simulink model "MDSC_PLL"  (R2018b)
settings: Solver=VariableStepAuto  StartTime=0.0  StopTime=10.0  RelTol=1e-3
libraries: simulink x1, powerlib_meascontrol x1, powerlib x1
(part 1 of 2)
settings Model: Creator=lokes  LastModifiedBy=lokes

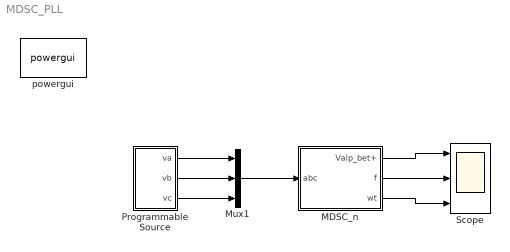
== system MDSC_PLL ==
  MDSC_n : Subsystem  mask{n=15, s=4, hr=1}
      mask prompts: n "MDSC Number (n)"; s "Selector (s): 1 for n= 6, 2 for n=9, 3 for n=12 and 4 for n=15"; hr "Required Component Extraction (hr)"
  Mux1 : Mux  Inputs=3
  Programmable Source : Subsystem  mask(CDSC - PLL){f=50, V=230}
      mask prompts: f "Fundamental grid frequency (f) in Hz"; V "Fundamental grid voltage (V) in RMS volts"
      mask help: Programmable source generates a signal with fundamental and odd harmonic signals upto 13th frequency component.
  Scope : Scope  NumInputPorts=3
  powergui : powerlib/powergui  Priority=1  SimulationMode=Discrete  SampleTime=10e-6  frequency=60  Iterations=50  frequencyindice=60  Pbase=100e6  ErrMax=1e-4  UnitsV=kV  UnitsW=MW  buscounter=0  FunctionMessages=off  echomessages=off  EnableUseOfTLC=off  CurrentSourceSwitches=off  DisableSnubberDevices=off  DisableRonSwitches=off  DisableVfSwitches=off  DisplayEquations=off  SolverType=Tustin  Interpol=off  ExternalGateDelay=off  methode=off  Ts=0  x0status=blocks  SPID=off  SwTol=0  HookPort=off  RestoreLinks=warning  ResistiveCurrentMeasurement=off  Frange=[0:2:500]  Ylog=off  Xlog=on  ShowGrid=off  save=off  variable=ZData  structure=0  ZoomFFT=off  StartTime=0.0  cycles=1  DisplayStyle=1  fundamental=60  FreqAxis=off  MaxFrequency=1000  frequencyindicesteady=1  RmsSteady=1  display=off
      settings: SourceProductName=Simscape Electrical
  wires:
  Programmable Source/1(va) -> Mux1/1
  Programmable Source/2(vb) -> Mux1/2
  Programmable Source/3(vc) -> Mux1/3
  Mux1/1 -> MDSC_n/1(abc)
  MDSC_n/1(Valp_bet+) -> Scope/1
  MDSC_n/2(f) -> Scope/2
  MDSC_n/3(wt) -> Scope/3

== system MDSC_PLL/MDSC_n ==
  abc : Inport
  3 : Constant  Value=0
  Demux : Demux  Outputs=3
  MDSC_n : Subsystem
  Mux6 : Mux  Inputs=2
  Mux7 : Mux  Inputs=2
  SRF-PLL1 : Subsystem
  abc to alpha-beta-Zero : Subsystem
      mask Display:
      | plot([0 1], [0,1])
      | text(0.15,0.7,'abc')
      | text(0.55, 0.3,'\alpha\beta0','texmode','on')
  Valp_bet+ : Outport
  f : Outport  Port=2
  wt : Outport  Port=3
  tag scope: f_pll_m3=global
  wires:
  abc/1 -> abc to alpha-beta-Zero/1(abc)
  abc to alpha-beta-Zero/1(al_be_0) -> Demux/1
  Demux/1 -> MDSC_n/1(Alpha)
  Demux/2 -> MDSC_n/2(Beta)
  MDSC_n/1(MDSC_n_alp) -> Mux6/1
  MDSC_n/2(MDSC_n_Bet) -> Mux6/2
  Mux6/1 -> Valp_bet+/1, Mux7/1
  3/1 -> Mux7/2
  Mux7/1 -> SRF-PLL1/1(al-be-0)
  SRF-PLL1/1(f) -> f/1, [f_pll_m3]
  SRF-PLL1/2(wt) -> wt/1

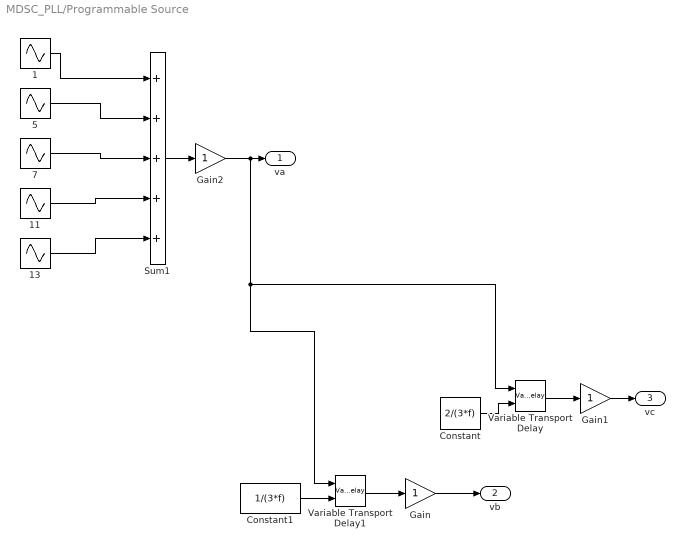
== system MDSC_PLL/Programmable Source ==
  1 : Sin  Amplitude=V*sqrt(2)  Frequency=2*pi*f  Phase=0*pi/2  SampleTime=0
  11 : Sin  Amplitude=V*sqrt(2)/11  Frequency=2*pi*11*f  Phase=0*pi/2  SampleTime=0
  13 : Sin  Amplitude=V*sqrt(2)/13  Frequency=2*pi*13*f  Phase=0*pi/2  SampleTime=0
  5 : Sin  Amplitude=V*sqrt(2)/5  Frequency=2*pi*5*f  Phase=0*pi/2  SampleTime=0
  7 : Sin  Amplitude=V*sqrt(2)/7  Frequency=2*pi*7*f  Phase=0*pi/2  SampleTime=0
  Constant : Constant  Value=2/(3*f)
  Constant1 : Constant  Value=1/(3*f)
  Gain : Gain
  Gain1 : Gain
  Gain2 : Gain
  Sum1 : Sum  Inputs=+++++
  Variable Transport Delay : VariableTransportDelay  VariableDelayType=Variable transport delay  MaximumDelay=10
  Variable Transport Delay1 : VariableTransportDelay  VariableDelayType=Variable transport delay  MaximumDelay=10
  va : Outport
  vb : Outport  Port=2
  vc : Outport  Port=3
  wires:
  Constant1/1 -> Variable Transport Delay1/2
  Constant/1 -> Variable Transport Delay/2
  Variable Transport Delay1/1 -> Gain/1
  Variable Transport Delay/1 -> Gain1/1
  Gain/1 -> vb/1
  Gain1/1 -> vc/1
  Sum1/1 -> Gain2/1
  Gain2/1 -> Variable Transport Delay1/1, Variable Transport Delay/1, va/1
  1/1 -> Sum1/1
  5/1 -> Sum1/2
  7/1 -> Sum1/3
  11/1 -> Sum1/4
  13/1 -> Sum1/5

== system MDSC_PLL/MDSC_n/MDSC_n ==
  Alpha : Inport
  Beta : Inport  Port=2
  DSC_Beta : Subsystem
  DSC_alpha : Subsystem
  MDSC_n_alp : Outport
  MDSC_n_Bet : Outport  Port=2
  wires:
  DSC_alpha/1(Out) -> MDSC_n_alp/1
  DSC_Beta/1(Out) -> MDSC_n_Bet/1
  Alpha/1 -> DSC_Beta/1(Alpha), DSC_alpha/1(Alpha)
  Beta/1 -> DSC_Beta/2(Beta), DSC_alpha/2(Beta)

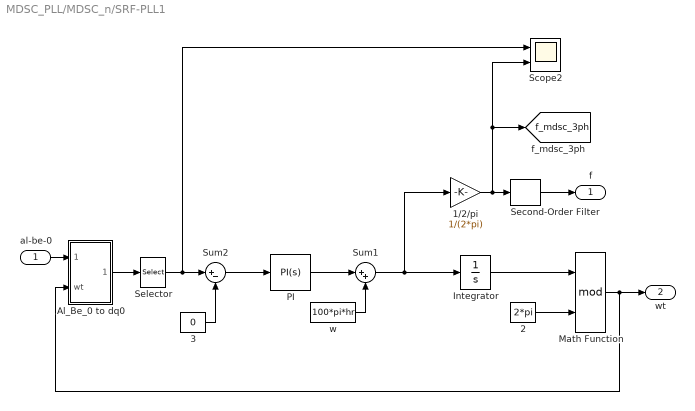
== system MDSC_PLL/MDSC_n/SRF-PLL1 ==
  al-be-0 : Inport
  1/2/pi : Gain  Gain=1/(2*pi)
  2 : Constant  Value=2*pi
  3 : Constant  Value=0
  Al_Be_0 to dq0 : Subsystem
      mask Display:
      | plot([0 1], [0,1])
      | port_label('input', 1, '\alpha\beta0','texmode','on')
      | port_label('input', 2, 'wt')
      | port_label('output', 1, 'dq0')
  Integrator : Integrator
  Math Function : Math  Operator=mod  SaturateOnIntegerOverflow=on
  "PI " : simulink/Continuous/PID Controller  Controller=PI  Form=Parallel  TimeDomain=Continuous-time  SampleTime=100e-6  IntegratorMethod=Forward Euler  FilterMethod=Forward Euler  ControllerParametersSource=internal  P=10  I=30  D=0  UseFilter=on  N=100  TunerSelectOption=Transfer Function Based (PID Tuner App)  InitialConditionSource=internal  InitialConditionForIntegrator=0  InitialConditionForFilter=0  DifferentiatorICPrevScaledInput=0  ExternalReset=none  TrackingMode=off  Kt=1  LimitOutput=off  UpperSaturationLimit=inf  LowerSaturationLimit=-inf  LinearizeAsGain=on  AntiWindupMode=none  Kb=1  POutMin=[]  POutMax=[]  IOutMin=[]  IOutMax=[]  DOutMin=[]  DOutMax=[]  NOutMin=[]  NOutMax=[]  SumOutMin=[]  SumOutMax=[]  SaturationOutMin=[]  SaturationOutMax=[]  PParamMin=[]  PParamMax=[]  IParamMin=[]  IParamMax=[]  DParamMin=[]  DParamMax=[]  NParamMin=[]  NParamMax=[]  KbParamMin=[]  KbParamMax=[]  KtParamMin=[]  KtParamMax=[]  KbOutMin=[]  KbOutMax=[]  KtOutMin=[]  KtOutMax=[]  IntegratorOutMin=[]  IntegratorOutMax=[]  FilterOutMin=[]  FilterOutMax=[]  SumI1OutMin=[]  SumI1OutMax=[]  SumI2OutMin=[]  SumI2OutMax=[]  SumI3OutMin=[]  SumI3OutMax=[]  SumI4OutMin=[]  SumI4OutMax=[]  SumDOutMin=[]  SumDOutMax=[]  DifferentiatorOutMin=[]  DifferentiatorOutMax=[]  FilterDiffOutCoefMin=[]  FilterDiffOutCoefMax=[]  ReciprocalOutMin=[]  ReciprocalOutMax=[]  SumDenOutMin=[]  SumDenOutMax=[]  SumNumOutMin=[]  SumNumOutMax=[]  DivideOutMin=[]  DivideOutMax=[]  IntegratorContinuousStateAttributes=''  IntegratorStateMustResolveToSignalObject=off  IntegratorRTWStateStorageClass=Auto  FilterContinuousStateAttributes=''  FilterStateMustResolveToSignalObject=off  FilterRTWStateStorageClass=Auto  ParallelPVariant=InternalParameters  IdealPVariant=Disabled  IVariant=InternalParameters  DVariant=Disabled  IntegratorVariant=Continuous  SatVariant=Disabled  AWVariant=Passthrough  PCopyVariant=Disabled  TRVariant=Disabled  FdbkBlocksVariant=Forward  IdealPFdbkVariant=Disabled  SatFdbkVariant=Disabled  DerivativeFilterVariant=Disabled  NVariant=Disabled  NCopyVariant=Disabled_SignalSpec  FilterICVariant=Disabled  IntegratorICVariant=InternalICs  ExternalResetVariant=Disabled  TRSumVariant=Passthrough  SumFdbkVariant=Disabled  SumVariant=Sum_PI
  Scope2 : Scope  NumInputPorts=2
  Second-Order Filter : powerlib_meascontrol/Filters/Second-Order Filter  FilterType=Lowpass  Fo=5  Zeta=0.707  Ts=0  Initialize=off  Vac_Init="[0,  0,  50]"  Vdc_Init=0  PlotResponse=off  FreqRange=[0, 500, 1]
      settings: SourceProductName=Simscape Electrical  SourceProductBaseCode=PS
  Selector : Selector  InputPortWidth=3  IndexOptions=Index vector (dialog)  Indices=1  OutputSizes=1
  Sum1 : Sum  Inputs=|++
  Sum2 : Sum  Inputs=|+-
  w : Constant  Value=100*pi*hr
  f : Outport
  wt : Outport  Port=2
  tag scope: f_mdsc_3ph=global
  wires:
  1/2/pi/1 -> Second-Order Filter/1, [f_mdsc_3ph], Scope2/2
  Math Function/1 -> Al_Be_0 to dq0/2(wt), wt/1
  Integrator/1 -> Math Function/1
  2/1 -> Math Function/2
  Sum1/1 -> Integrator/1, 1/2/pi/1
  w/1 -> Sum1/2
  "PI "/1 -> Sum1/1
  Sum2/1 -> "PI "/1
  al-be-0/1 -> Al_Be_0 to dq0/1(Al_Be_0)
  3/1 -> Sum2/2
  Al_Be_0 to dq0/1(dq0) -> Selector/1
  Selector/1 -> Sum2/1, Scope2/1
  Second-Order Filter/1 -> f/1

== system MDSC_PLL/MDSC_n/abc to alpha-beta-Zero ==
  abc : Inport
  Gain1 : Gain  Gain=(2/3)  SaturateOnIntegerOverflow=on  OutDataTypeStr=Inherit: Same as input  ParamDataTypeStr=Inherit: Same as input
  Gain3 : Gain  Gain="[ 1   -1/2   -1/2; 0   sqrt(3)/2   -sqrt(3)/2; 1/(2)  1/(2)  1/(2) ]"  Multiplication=Matrix(K*u) (u vector)  SaturateOnIntegerOverflow=on  OutDataTypeStr=Inherit: Same as input  ParamDataTypeStr=Inherit: Same as input
  al_be_0 : Outport
  wires:
  Gain3/1 -> Gain1/1
  Gain1/1 -> al_be_0/1
  abc/1 -> Gain3/1

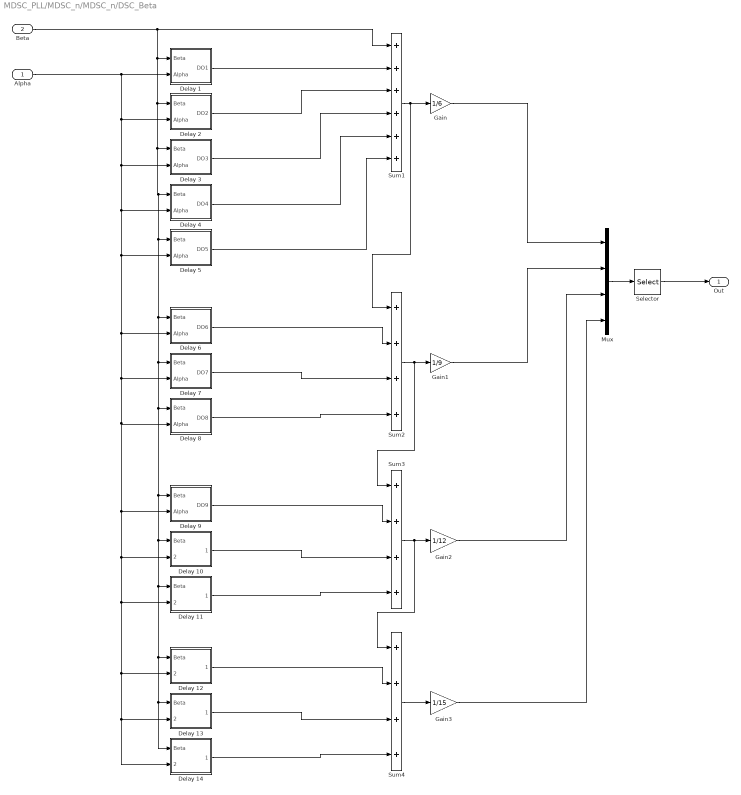
== system MDSC_PLL/MDSC_n/MDSC_n/DSC_Beta ==
  Alpha : Inport
  Beta : Inport  Port=2
  Delay 1 : Subsystem
  Delay 10 : Subsystem
  Delay 11 : Subsystem
  Delay 12 : Subsystem
  Delay 13 : Subsystem
  Delay 14 : Subsystem
  Delay 2 : Subsystem
  Delay 3 : Subsystem
  Delay 4 : Subsystem
  Delay 5 : Subsystem
  Delay 6 : Subsystem
  Delay 7 : Subsystem
  Delay 8 : Subsystem
  Delay 9 : Subsystem
  Gain : Gain  Gain=1/6
  Gain1 : Gain  Gain=1/9
  Gain2 : Gain  Gain=1/12
  Gain3 : Gain  Gain=1/15
  Mux : Mux
  Selector : Selector  InputPortWidth=4  IndexOptions=Index vector (dialog)  Indices=s  OutputSizes=1
  Sum1 : Sum  Inputs=++++++
  Sum2 : Sum  Inputs=++++
  Sum3 : Sum  Inputs=++++
  Sum4 : Sum  Inputs=++++
  Out : Outport
  wires:
  Selector/1 -> Out/1
  Gain3/1 -> Mux/4
  Gain2/1 -> Mux/3
  Gain1/1 -> Mux/2
  Gain/1 -> Mux/1
  Mux/1 -> Selector/1
  Delay 14/1(DO14) -> Sum4/4
  Delay 13/1(DO13) -> Sum4/3
  Delay 12/1(DO12) -> Sum4/2
  Alpha/1 -> Delay 1/2(Alpha), Delay 2/2(Alpha), Delay 3/2(Alpha), Delay 4/2(Alpha), Delay 5/2(Alpha), Delay 6/2(Alpha), Delay 7/2(Alpha), Delay 8/2(Alpha), Delay 9/2(Alpha), Delay 10/2(Alpha), Delay 11/2(Alpha), Delay 14/2(Alpha), Delay 13/2(Alpha), Delay 12/2(Alpha)
  Sum4/1 -> Gain3/1
  Beta/1 -> Sum1/1, Delay 1/1(Beta), Delay 3/1(Beta), Delay 4/1(Beta), Delay 6/1(Beta), Delay 7/1(Beta), Delay 8/1(Beta), Delay 9/1(Beta), Delay 10/1(Beta), Delay 11/1(Beta), Delay 14/1(Beta), Delay 13/1(Beta), Delay 12/1(Beta), Delay 5/1(Beta), Delay 2/1(Beta)
  Sum3/1 -> Gain2/1, Sum4/1
  Delay 11/1(DO11) -> Sum3/4
  Delay 10/1(DO10) -> Sum3/3
  Delay 9/1(DO9) -> Sum3/2
  Delay 8/1(DO8) -> Sum2/4
  Delay 7/1(DO7) -> Sum2/3
  Delay 6/1(DO6) -> Sum2/2
  Sum2/1 -> Gain1/1, Sum3/1
  Delay 5/1(DO5) -> Sum1/6
  Delay 4/1(DO4) -> Sum1/5
  Delay 3/1(DO3) -> Sum1/4
  Delay 2/1(DO2) -> Sum1/3
  Delay 1/1(DO1) -> Sum1/2
  Sum1/1 -> Gain/1, Sum2/1

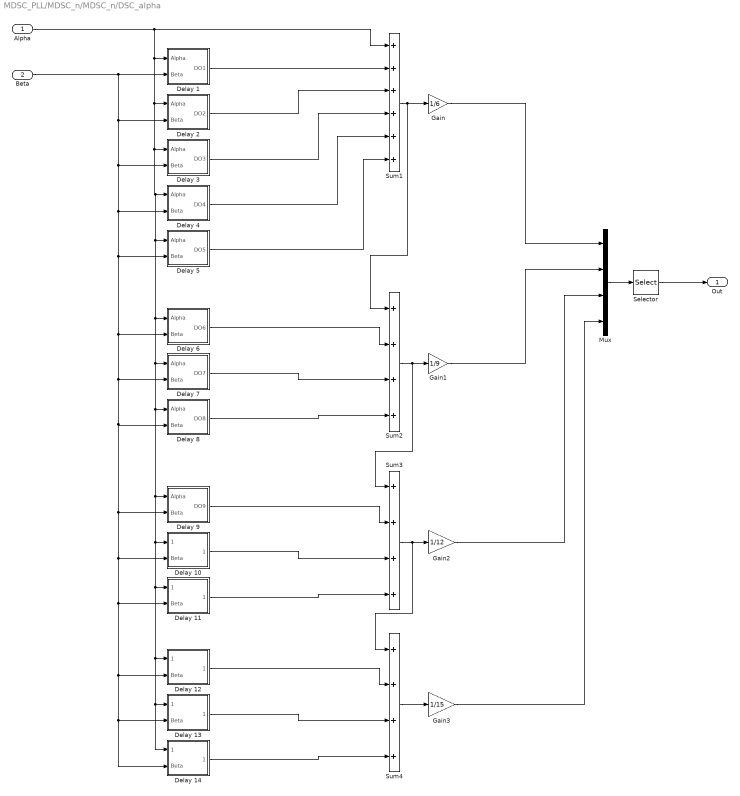
== system MDSC_PLL/MDSC_n/MDSC_n/DSC_alpha ==
  Alpha : Inport
  Beta : Inport  Port=2
  Delay 1 : Subsystem
  Delay 10 : Subsystem
  Delay 11 : Subsystem
  Delay 12 : Subsystem
  Delay 13 : Subsystem
  Delay 14 : Subsystem
  Delay 2 : Subsystem
  Delay 3 : Subsystem
  Delay 4 : Subsystem
  Delay 5 : Subsystem
  Delay 6 : Subsystem
  Delay 7 : Subsystem
  Delay 8 : Subsystem
  Delay 9 : Subsystem
  Gain : Gain  Gain=1/6
  Gain1 : Gain  Gain=1/9
  Gain2 : Gain  Gain=1/12
  Gain3 : Gain  Gain=1/15
  Mux : Mux
  Selector : Selector  InputPortWidth=4  IndexOptions=Index vector (dialog)  Indices=s  OutputSizes=1
  Sum1 : Sum  Inputs=++++++
  Sum2 : Sum  Inputs=++++
  Sum3 : Sum  Inputs=++++
  Sum4 : Sum  Inputs=++++
  Out : Outport
  wires:
  Sum1/1 -> Sum2/1, Gain/1
  Delay 1/1(DO1) -> Sum1/2
  Delay 2/1(DO2) -> Sum1/3
  Delay 3/1(DO3) -> Sum1/4
  Delay 4/1(DO4) -> Sum1/5
  Delay 5/1(DO5) -> Sum1/6
  Sum2/1 -> Sum3/1, Gain1/1
  Delay 6/1(DO6) -> Sum2/2
  Delay 7/1(DO7) -> Sum2/3
  Delay 8/1(DO8) -> Sum2/4
  Delay 9/1(DO9) -> Sum3/2
  Delay 10/1(DO10) -> Sum3/3
  Delay 11/1(DO11) -> Sum3/4
  Sum3/1 -> Sum4/1, Gain2/1
  Alpha/1 -> Delay 2/1(Alpha), Delay 5/1(Alpha), Delay 12/1(Alpha), Delay 13/1(Alpha), Delay 14/1(Alpha), Delay 11/1(Alpha), Delay 10/1(Alpha), Delay 9/1(Alpha), Delay 8/1(Alpha), Delay 7/1(Alpha), Delay 6/1(Alpha), Delay 4/1(Alpha), Delay 3/1(Alpha), Delay 1/1(Alpha), Sum1/1
  Sum4/1 -> Gain3/1
  Beta/1 -> Delay 12/2(Beta), Delay 13/2(Beta), Delay 14/2(Beta), Delay 11/2(Beta), Delay 10/2(Beta), Delay 9/2(Beta), Delay 8/2(Beta), Delay 7/2(Beta), Delay 6/2(Beta), Delay 5/2(Beta), Delay 4/2(Beta), Delay 3/2(Beta), Delay 2/2(Beta), Delay 1/2(Beta)
  Delay 12/1(DO12) -> Sum4/2
  Delay 13/1(DO13) -> Sum4/3
  Delay 14/1(DO14) -> Sum4/4
  Mux/1 -> Selector/1
  Gain/1 -> Mux/1
  Gain1/1 -> Mux/2
  Gain2/1 -> Mux/3
  Gain3/1 -> Mux/4
  Selector/1 -> Out/1

== system MDSC_PLL/MDSC_n/SRF-PLL1/Al_Be_0 to dq0 ==
  Al_Be_0 : Inport
  wt : Inport  Port=2
  Fcn : Fcn  Expr=u[1]*cos(u[4]) + u[2]*sin(u[4])
  Fcn1 : Fcn  Expr=-u[1]*sin(u[4]) + u[2]*cos(u[4])
  Fcn2 : Fcn  Expr=u[3]
  Mux1 : Mux  Inputs=[3 1]
  Mux2 : Mux  Inputs=3
  dq0 : Outport
  wires:
  Mux1/1 -> Fcn/1, Fcn2/1, Fcn1/1
  Fcn1/1 -> Mux2/2
  wt/1 -> Mux1/2
  Mux2/1 -> dq0/1
  Al_Be_0/1 -> Mux1/1
  Fcn2/1 -> Mux2/3
  Fcn/1 -> Mux2/1

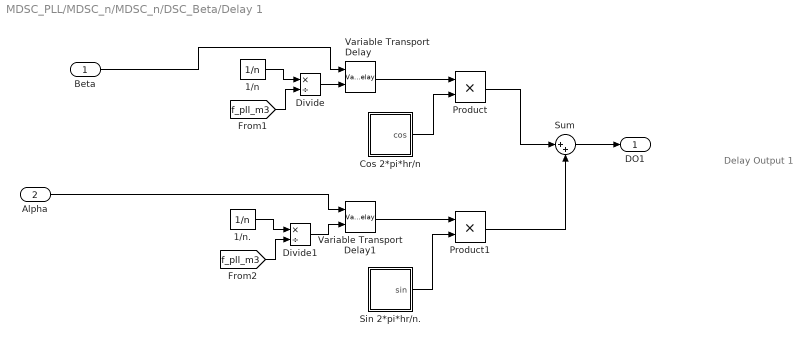
== system MDSC_PLL/MDSC_n/MDSC_n/DSC_Beta/Delay 1 ==
  note: Delay Output 1
  Beta : Inport
  Alpha : Inport  Port=2
  1/n : Constant  Value=1/n
  1/n. : Constant  Value=1/n
  Cos 2*pi*hr/n : Subsystem
  Divide : Product  Inputs=*/
  Divide1 : Product  Inputs=*/
  Product : Product
  Product1 : Product
  Sin 2*pi*hr/n. : Subsystem
  Sum : Sum  Inputs=|++
  Variable Transport Delay : VariableTransportDelay  VariableDelayType=Variable transport delay  MaximumDelay=10
  Variable Transport Delay1 : VariableTransportDelay  VariableDelayType=Variable transport delay  MaximumDelay=10
  DO1 : Outport
  wires:
  Sum/1 -> DO1/1
  Product1/1 -> Sum/2
  Product/1 -> Sum/1
  Beta/1 -> Variable Transport Delay/1
  1/n/1 -> Divide/1
  [f_pll_m3] -> Divide/2
  [f_pll_m3] -> Divide1/2
  1/n./1 -> Divide1/1
  Divide1/1 -> Variable Transport Delay1/2
  Divide/1 -> Variable Transport Delay/2
  Sin 2*pi*hr/n./1(sin) -> Product1/2
  Alpha/1 -> Variable Transport Delay1/1
  Variable Transport Delay1/1 -> Product1/1
  Variable Transport Delay/1 -> Product/1
  Cos 2*pi*hr/n/1(cos) -> Product/2

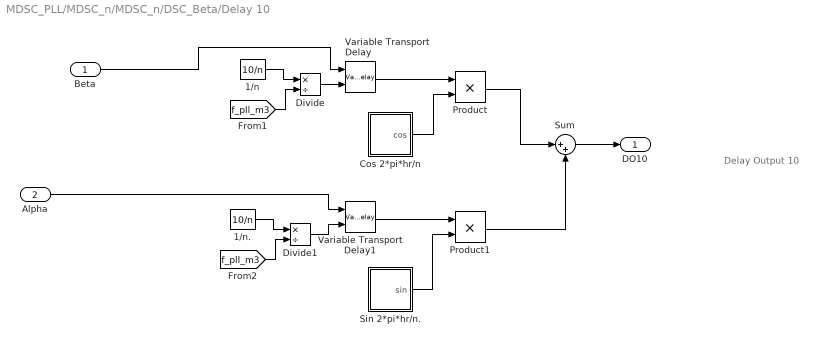
== system MDSC_PLL/MDSC_n/MDSC_n/DSC_Beta/Delay 10 ==
  note: Delay Output 10
  Beta : Inport
  Alpha : Inport  Port=2
  1/n : Constant  Value=10/n
  1/n. : Constant  Value=10/n
  Cos 2*pi*hr/n : Subsystem
  Divide : Product  Inputs=*/
  Divide1 : Product  Inputs=*/
  Product : Product
  Product1 : Product
  Sin 2*pi*hr/n. : Subsystem
  Sum : Sum  Inputs=|++
  Variable Transport Delay : VariableTransportDelay  VariableDelayType=Variable transport delay  MaximumDelay=10
  Variable Transport Delay1 : VariableTransportDelay  VariableDelayType=Variable transport delay  MaximumDelay=10
  DO10 : Outport
  wires:
  Cos 2*pi*hr/n/1(cos) -> Product/2
  Variable Transport Delay/1 -> Product/1
  Variable Transport Delay1/1 -> Product1/1
  Alpha/1 -> Variable Transport Delay1/1
  Sin 2*pi*hr/n./1(sin) -> Product1/2
  Divide/1 -> Variable Transport Delay/2
  Divide1/1 -> Variable Transport Delay1/2
  1/n./1 -> Divide1/1
  [f_pll_m3] -> Divide1/2
  [f_pll_m3] -> Divide/2
  1/n/1 -> Divide/1
  Beta/1 -> Variable Transport Delay/1
  Product/1 -> Sum/1
  Product1/1 -> Sum/2
  Sum/1 -> DO10/1

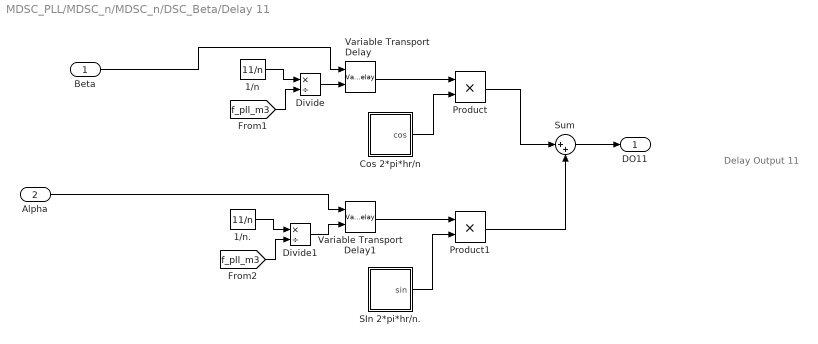
== system MDSC_PLL/MDSC_n/MDSC_n/DSC_Beta/Delay 11 ==
  note: Delay Output 11
  Beta : Inport
  Alpha : Inport  Port=2
  1/n : Constant  Value=11/n
  1/n. : Constant  Value=11/n
  Cos 2*pi*hr/n : Subsystem
  Divide : Product  Inputs=*/
  Divide1 : Product  Inputs=*/
  Product : Product
  Product1 : Product
  SIn 2*pi*hr/n. : Subsystem
  Sum : Sum  Inputs=|++
  Variable Transport Delay : VariableTransportDelay  VariableDelayType=Variable transport delay  MaximumDelay=10
  Variable Transport Delay1 : VariableTransportDelay  VariableDelayType=Variable transport delay  MaximumDelay=10
  DO11 : Outport
  wires:
  Sum/1 -> DO11/1
  Product1/1 -> Sum/2
  Product/1 -> Sum/1
  Beta/1 -> Variable Transport Delay/1
  1/n/1 -> Divide/1
  [f_pll_m3] -> Divide/2
  [f_pll_m3] -> Divide1/2
  1/n./1 -> Divide1/1
  Divide1/1 -> Variable Transport Delay1/2
  Divide/1 -> Variable Transport Delay/2
  SIn 2*pi*hr/n./1(sin) -> Product1/2
  Alpha/1 -> Variable Transport Delay1/1
  Variable Transport Delay1/1 -> Product1/1
  Variable Transport Delay/1 -> Product/1
  Cos 2*pi*hr/n/1(cos) -> Product/2

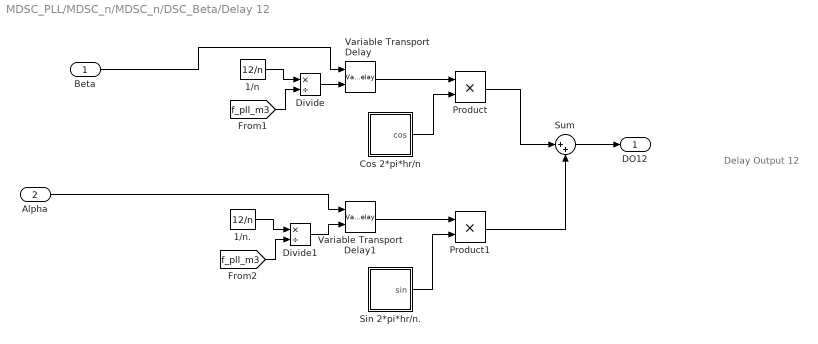
== system MDSC_PLL/MDSC_n/MDSC_n/DSC_Beta/Delay 12 ==
  note: Delay Output 12
  Beta : Inport
  Alpha : Inport  Port=2
  1/n : Constant  Value=12/n
  1/n. : Constant  Value=12/n
  Cos 2*pi*hr/n : Subsystem
  Divide : Product  Inputs=*/
  Divide1 : Product  Inputs=*/
  Product : Product
  Product1 : Product
  Sin 2*pi*hr/n. : Subsystem
  Sum : Sum  Inputs=|++
  Variable Transport Delay : VariableTransportDelay  VariableDelayType=Variable transport delay  MaximumDelay=10
  Variable Transport Delay1 : VariableTransportDelay  VariableDelayType=Variable transport delay  MaximumDelay=10
  DO12 : Outport
  wires:
  Cos 2*pi*hr/n/1(cos) -> Product/2
  Variable Transport Delay/1 -> Product/1
  Variable Transport Delay1/1 -> Product1/1
  Alpha/1 -> Variable Transport Delay1/1
  Sin 2*pi*hr/n./1(sin) -> Product1/2
  Divide/1 -> Variable Transport Delay/2
  Divide1/1 -> Variable Transport Delay1/2
  1/n./1 -> Divide1/1
  [f_pll_m3] -> Divide1/2
  [f_pll_m3] -> Divide/2
  1/n/1 -> Divide/1
  Beta/1 -> Variable Transport Delay/1
  Product/1 -> Sum/1
  Product1/1 -> Sum/2
  Sum/1 -> DO12/1

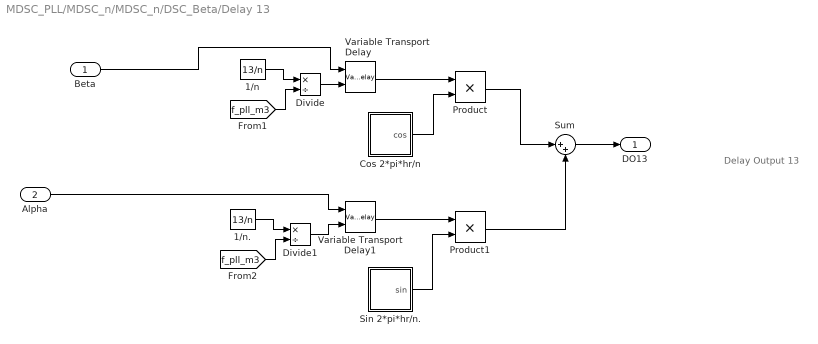
== system MDSC_PLL/MDSC_n/MDSC_n/DSC_Beta/Delay 13 ==
  note: Delay Output 13
  Beta : Inport
  Alpha : Inport  Port=2
  1/n : Constant  Value=13/n
  1/n. : Constant  Value=13/n
  Cos 2*pi*hr/n : Subsystem
  Divide : Product  Inputs=*/
  Divide1 : Product  Inputs=*/
  Product : Product
  Product1 : Product
  Sin 2*pi*hr/n. : Subsystem
  Sum : Sum  Inputs=|++
  Variable Transport Delay : VariableTransportDelay  VariableDelayType=Variable transport delay  MaximumDelay=10
  Variable Transport Delay1 : VariableTransportDelay  VariableDelayType=Variable transport delay  MaximumDelay=10
  DO13 : Outport
  wires:
  Sum/1 -> DO13/1
  Product1/1 -> Sum/2
  Product/1 -> Sum/1
  Beta/1 -> Variable Transport Delay/1
  1/n/1 -> Divide/1
  [f_pll_m3] -> Divide/2
  [f_pll_m3] -> Divide1/2
  1/n./1 -> Divide1/1
  Divide1/1 -> Variable Transport Delay1/2
  Divide/1 -> Variable Transport Delay/2
  Sin 2*pi*hr/n./1(sin) -> Product1/2
  Alpha/1 -> Variable Transport Delay1/1
  Variable Transport Delay1/1 -> Product1/1
  Variable Transport Delay/1 -> Product/1
  Cos 2*pi*hr/n/1(cos) -> Product/2

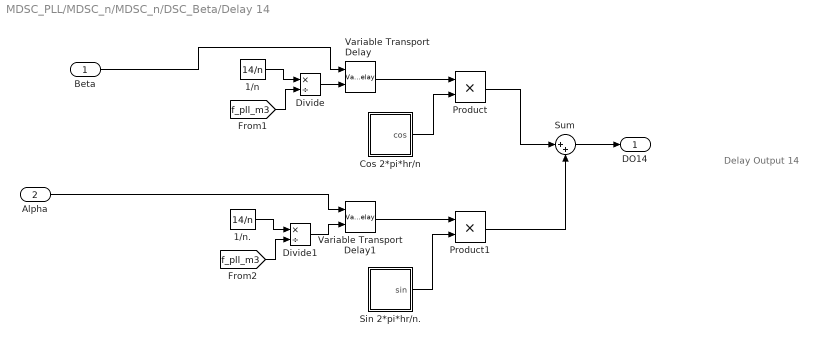
== system MDSC_PLL/MDSC_n/MDSC_n/DSC_Beta/Delay 14 ==
  note: Delay Output 14
  Beta : Inport
  Alpha : Inport  Port=2
  1/n : Constant  Value=14/n
  1/n. : Constant  Value=14/n
  Cos 2*pi*hr/n : Subsystem
  Divide : Product  Inputs=*/
  Divide1 : Product  Inputs=*/
  Product : Product
  Product1 : Product
  Sin 2*pi*hr/n. : Subsystem
  Sum : Sum  Inputs=|++
  Variable Transport Delay : VariableTransportDelay  VariableDelayType=Variable transport delay  MaximumDelay=10
  Variable Transport Delay1 : VariableTransportDelay  VariableDelayType=Variable transport delay  MaximumDelay=10
  DO14 : Outport
  wires:
  Cos 2*pi*hr/n/1(cos) -> Product/2
  Variable Transport Delay/1 -> Product/1
  Variable Transport Delay1/1 -> Product1/1
  Alpha/1 -> Variable Transport Delay1/1
  Sin 2*pi*hr/n./1(sin) -> Product1/2
  Divide/1 -> Variable Transport Delay/2
  Divide1/1 -> Variable Transport Delay1/2
  1/n./1 -> Divide1/1
  [f_pll_m3] -> Divide1/2
  [f_pll_m3] -> Divide/2
  1/n/1 -> Divide/1
  Beta/1 -> Variable Transport Delay/1
  Product/1 -> Sum/1
  Product1/1 -> Sum/2
  Sum/1 -> DO14/1

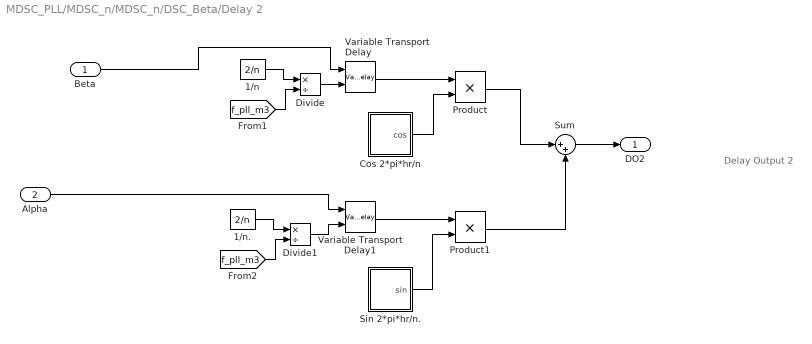
== system MDSC_PLL/MDSC_n/MDSC_n/DSC_Beta/Delay 2 ==
  note: Delay Output 2
  Beta : Inport
  Alpha : Inport  Port=2
  1/n : Constant  Value=2/n
  1/n. : Constant  Value=2/n
  Cos 2*pi*hr/n : Subsystem
  Divide : Product  Inputs=*/
  Divide1 : Product  Inputs=*/
  Product : Product
  Product1 : Product
  Sin 2*pi*hr/n. : Subsystem
  Sum : Sum  Inputs=|++
  Variable Transport Delay : VariableTransportDelay  VariableDelayType=Variable transport delay  MaximumDelay=10
  Variable Transport Delay1 : VariableTransportDelay  VariableDelayType=Variable transport delay  MaximumDelay=10
  DO2 : Outport
  wires:
  Cos 2*pi*hr/n/1(cos) -> Product/2
  Variable Transport Delay/1 -> Product/1
  Variable Transport Delay1/1 -> Product1/1
  Alpha/1 -> Variable Transport Delay1/1
  Sin 2*pi*hr/n./1(sin) -> Product1/2
  Divide/1 -> Variable Transport Delay/2
  Divide1/1 -> Variable Transport Delay1/2
  1/n./1 -> Divide1/1
  [f_pll_m3] -> Divide1/2
  [f_pll_m3] -> Divide/2
  1/n/1 -> Divide/1
  Beta/1 -> Variable Transport Delay/1
  Product/1 -> Sum/1
  Product1/1 -> Sum/2
  Sum/1 -> DO2/1

== system MDSC_PLL/MDSC_n/MDSC_n/DSC_Beta/Delay 3 ==
  note: Delay Output 3
  Beta : Inport
  Alpha : Inport  Port=2
  1/n : Constant  Value=3/n
  1/n. : Constant  Value=3/n
  Cos 2*pi*hr/n : Subsystem
  Divide : Product  Inputs=*/
  Divide1 : Product  Inputs=*/
  Product : Product
  Product1 : Product
  Sin 2*pi*hr/n. : Subsystem
  Sum : Sum  Inputs=|++
  Variable Transport Delay : VariableTransportDelay  VariableDelayType=Variable transport delay  MaximumDelay=10
  Variable Transport Delay1 : VariableTransportDelay  VariableDelayType=Variable transport delay  MaximumDelay=10
  DO3 : Outport
  wires:
  Sum/1 -> DO3/1
  Product1/1 -> Sum/2
  Product/1 -> Sum/1
  Beta/1 -> Variable Transport Delay/1
  1/n/1 -> Divide/1
  [f_pll_m3] -> Divide/2
  [f_pll_m3] -> Divide1/2
  1/n./1 -> Divide1/1
  Divide1/1 -> Variable Transport Delay1/2
  Divide/1 -> Variable Transport Delay/2
  Sin 2*pi*hr/n./1(sin) -> Product1/2
  Alpha/1 -> Variable Transport Delay1/1
  Variable Transport Delay1/1 -> Product1/1
  Variable Transport Delay/1 -> Product/1
  Cos 2*pi*hr/n/1(cos) -> Product/2

== system MDSC_PLL/MDSC_n/MDSC_n/DSC_Beta/Delay 4 ==
  note: Delay Output 4
  Beta : Inport
  Alpha : Inport  Port=2
  1/n : Constant  Value=4/n
  1/n. : Constant  Value=4/n
  Cos 2*pi*hr/n : Subsystem
  Divide : Product  Inputs=*/
  Divide1 : Product  Inputs=*/
  Product : Product
  Product1 : Product
  Sin 2*pi*hr/n. : Subsystem
  Sum : Sum  Inputs=|++
  Variable Transport Delay : VariableTransportDelay  VariableDelayType=Variable transport delay  MaximumDelay=10
  Variable Transport Delay1 : VariableTransportDelay  VariableDelayType=Variable transport delay  MaximumDelay=10
  DO4 : Outport
  wires:
  Cos 2*pi*hr/n/1(cos) -> Product/2
  Variable Transport Delay/1 -> Product/1
  Variable Transport Delay1/1 -> Product1/1
  Alpha/1 -> Variable Transport Delay1/1
  Sin 2*pi*hr/n./1(sin) -> Product1/2
  Divide/1 -> Variable Transport Delay/2
  Divide1/1 -> Variable Transport Delay1/2
  1/n./1 -> Divide1/1
  [f_pll_m3] -> Divide1/2
  [f_pll_m3] -> Divide/2
  1/n/1 -> Divide/1
  Beta/1 -> Variable Transport Delay/1
  Product/1 -> Sum/1
  Product1/1 -> Sum/2
  Sum/1 -> DO4/1

== system MDSC_PLL/MDSC_n/MDSC_n/DSC_Beta/Delay 5 ==
  note: Delay Output 5
  Beta : Inport
  Alpha : Inport  Port=2
  1/n : Constant  Value=5/n
  1/n. : Constant  Value=5/n
  Cos 2*pi*hr/n : Subsystem
  Divide : Product  Inputs=*/
  Divide1 : Product  Inputs=*/
  Product : Product
  Product1 : Product
  Sin 2*pi*hr/n. : Subsystem
  Sum : Sum  Inputs=|++
  Variable Transport Delay : VariableTransportDelay  VariableDelayType=Variable transport delay  MaximumDelay=10
  Variable Transport Delay1 : VariableTransportDelay  VariableDelayType=Variable transport delay  MaximumDelay=10
  DO5 : Outport
  wires:
  Sum/1 -> DO5/1
  Product1/1 -> Sum/2
  Product/1 -> Sum/1
  Beta/1 -> Variable Transport Delay/1
  1/n/1 -> Divide/1
  [f_pll_m3] -> Divide/2
  [f_pll_m3] -> Divide1/2
  1/n./1 -> Divide1/1
  Divide1/1 -> Variable Transport Delay1/2
  Divide/1 -> Variable Transport Delay/2
  Sin 2*pi*hr/n./1(sin) -> Product1/2
  Alpha/1 -> Variable Transport Delay1/1
  Variable Transport Delay1/1 -> Product1/1
  Variable Transport Delay/1 -> Product/1
  Cos 2*pi*hr/n/1(cos) -> Product/2

== system MDSC_PLL/MDSC_n/MDSC_n/DSC_Beta/Delay 6 ==
  note: Delay Output 6
  Beta : Inport
  Alpha : Inport  Port=2
  1/n : Constant  Value=6/n
  1/n. : Constant  Value=6/n
  Cos 2*pi*hr/n : Subsystem
  Divide : Product  Inputs=*/
  Divide1 : Product  Inputs=*/
  Product : Product
  Product1 : Product
  Sin 2*pi*hr/n. : Subsystem
  Sum : Sum  Inputs=|++
  Variable Transport Delay : VariableTransportDelay  VariableDelayType=Variable transport delay  MaximumDelay=10
  Variable Transport Delay1 : VariableTransportDelay  VariableDelayType=Variable transport delay  MaximumDelay=10
  DO6 : Outport
  wires:
  Sum/1 -> DO6/1
  Product1/1 -> Sum/2
  Product/1 -> Sum/1
  Beta/1 -> Variable Transport Delay/1
  1/n/1 -> Divide/1
  [f_pll_m3] -> Divide/2
  [f_pll_m3] -> Divide1/2
  1/n./1 -> Divide1/1
  Divide1/1 -> Variable Transport Delay1/2
  Divide/1 -> Variable Transport Delay/2
  Sin 2*pi*hr/n./1(sin) -> Product1/2
  Alpha/1 -> Variable Transport Delay1/1
  Variable Transport Delay1/1 -> Product1/1
  Variable Transport Delay/1 -> Product/1
  Cos 2*pi*hr/n/1(cos) -> Product/2

== system MDSC_PLL/MDSC_n/MDSC_n/DSC_Beta/Delay 7 ==
  note: Delay Output 7
  Beta : Inport
  Alpha : Inport  Port=2
  1/n : Constant  Value=7/n
  1/n. : Constant  Value=7/n
  Cos 2*pi*hr/n : Subsystem
  Divide : Product  Inputs=*/
  Divide1 : Product  Inputs=*/
  Product : Product
  Product1 : Product
  Sin 2*pi*hr/n. : Subsystem
  Sum : Sum  Inputs=|++
  Variable Transport Delay : VariableTransportDelay  VariableDelayType=Variable transport delay  MaximumDelay=10
  Variable Transport Delay1 : VariableTransportDelay  VariableDelayType=Variable transport delay  MaximumDelay=10
  DO7 : Outport
  wires:
  Cos 2*pi*hr/n/1(cos) -> Product/2
  Variable Transport Delay/1 -> Product/1
  Variable Transport Delay1/1 -> Product1/1
  Alpha/1 -> Variable Transport Delay1/1
  Sin 2*pi*hr/n./1(sin) -> Product1/2
  Divide/1 -> Variable Transport Delay/2
  Divide1/1 -> Variable Transport Delay1/2
  1/n./1 -> Divide1/1
  [f_pll_m3] -> Divide1/2
  [f_pll_m3] -> Divide/2
  1/n/1 -> Divide/1
  Beta/1 -> Variable Transport Delay/1
  Product/1 -> Sum/1
  Product1/1 -> Sum/2
  Sum/1 -> DO7/1

== system MDSC_PLL/MDSC_n/MDSC_n/DSC_Beta/Delay 8 ==
  note: Delay Output 8
  Beta : Inport
  Alpha : Inport  Port=2
  1/n : Constant  Value=8/n
  1/n. : Constant  Value=8/n
  Cos 2*pi*hr/n : Subsystem
  Divide : Product  Inputs=*/
  Divide1 : Product  Inputs=*/
  Product : Product
  Product1 : Product
  Sin 2*pi*hr/n. : Subsystem
  Sum : Sum  Inputs=|++
  Variable Transport Delay : VariableTransportDelay  VariableDelayType=Variable transport delay  MaximumDelay=10
  Variable Transport Delay1 : VariableTransportDelay  VariableDelayType=Variable transport delay  MaximumDelay=10
  DO8 : Outport
  wires:
  Sum/1 -> DO8/1
  Product1/1 -> Sum/2
  Product/1 -> Sum/1
  Beta/1 -> Variable Transport Delay/1
  1/n/1 -> Divide/1
  [f_pll_m3] -> Divide/2
  [f_pll_m3] -> Divide1/2
  1/n./1 -> Divide1/1
  Divide1/1 -> Variable Transport Delay1/2
  Divide/1 -> Variable Transport Delay/2
  Sin 2*pi*hr/n./1(sin) -> Product1/2
  Alpha/1 -> Variable Transport Delay1/1
  Variable Transport Delay1/1 -> Product1/1
  Variable Transport Delay/1 -> Product/1
  Cos 2*pi*hr/n/1(cos) -> Product/2

== system MDSC_PLL/MDSC_n/MDSC_n/DSC_Beta/Delay 9 ==
  note: Delay Output 9
  Beta : Inport
  Alpha : Inport  Port=2
  1/n : Constant  Value=9/n
  1/n. : Constant  Value=9/n
  Cos 2*pi*hr/n : Subsystem
  Divide : Product  Inputs=*/
  Divide1 : Product  Inputs=*/
  Product : Product
  Product1 : Product
  Sin 2*pi*hr/n. : Subsystem
  Sum : Sum  Inputs=|++
  Variable Transport Delay : VariableTransportDelay  VariableDelayType=Variable transport delay  MaximumDelay=10
  Variable Transport Delay1 : VariableTransportDelay  VariableDelayType=Variable transport delay  MaximumDelay=10
  DO9 : Outport
  wires:
  Sum/1 -> DO9/1
  Product1/1 -> Sum/2
  Product/1 -> Sum/1
  Beta/1 -> Variable Transport Delay/1
  1/n/1 -> Divide/1
  [f_pll_m3] -> Divide/2
  [f_pll_m3] -> Divide1/2
  1/n./1 -> Divide1/1
  Divide1/1 -> Variable Transport Delay1/2
  Divide/1 -> Variable Transport Delay/2
  Sin 2*pi*hr/n./1(sin) -> Product1/2
  Alpha/1 -> Variable Transport Delay1/1
  Variable Transport Delay1/1 -> Product1/1
  Variable Transport Delay/1 -> Product/1
  Cos 2*pi*hr/n/1(cos) -> Product/2

== system MDSC_PLL/MDSC_n/MDSC_n/DSC_alpha/Delay 1 ==
  note: Delay Output 1
  Alpha : Inport
  Beta : Inport  Port=2
  1/n : Constant  Value=1/n
  1/n. : Constant  Value=1/n
  Cos 2*pi*hr/n : Subsystem
  Divide : Product  Inputs=*/
  Divide1 : Product  Inputs=*/
  Product : Product
  Product1 : Product
  Sin 2*pi*hr/n. : Subsystem
  Sum : Sum  Inputs=|+-
  Variable Transport Delay : VariableTransportDelay  VariableDelayType=Variable transport delay  MaximumDelay=10
  Variable Transport Delay1 : VariableTransportDelay  VariableDelayType=Variable transport delay  MaximumDelay=10
  DO1 : Outport
  wires:
  Cos 2*pi*hr/n/1(cos) -> Product/2
  Variable Transport Delay/1 -> Product/1
  Variable Transport Delay1/1 -> Product1/1
  Beta/1 -> Variable Transport Delay1/1
  Sin 2*pi*hr/n./1(sin) -> Product1/2
  Divide/1 -> Variable Transport Delay/2
  Divide1/1 -> Variable Transport Delay1/2
  1/n./1 -> Divide1/1
  [f_pll_m3] -> Divide1/2
  [f_pll_m3] -> Divide/2
  1/n/1 -> Divide/1
  Alpha/1 -> Variable Transport Delay/1
  Product/1 -> Sum/1
  Product1/1 -> Sum/2
  Sum/1 -> DO1/1

== system MDSC_PLL/MDSC_n/MDSC_n/DSC_alpha/Delay 10 ==
  note: Delay Output 10
  Alpha : Inport
  Beta : Inport  Port=2
  1/n : Constant  Value=10/n
  1/n. : Constant  Value=10/n
  Cos 2*pi*hr/n : Subsystem
  Divide : Product  Inputs=*/
  Divide1 : Product  Inputs=*/
  Product : Product
  Product1 : Product
  Sin 2*pi*hr/n. : Subsystem
  Sum : Sum  Inputs=|+-
  Variable Transport Delay : VariableTransportDelay  VariableDelayType=Variable transport delay  MaximumDelay=10
  Variable Transport Delay1 : VariableTransportDelay  VariableDelayType=Variable transport delay  MaximumDelay=10
  DO10 : Outport
  wires:
  Sum/1 -> DO10/1
  Product1/1 -> Sum/2
  Product/1 -> Sum/1
  Alpha/1 -> Variable Transport Delay/1
  1/n/1 -> Divide/1
  [f_pll_m3] -> Divide/2
  [f_pll_m3] -> Divide1/2
  1/n./1 -> Divide1/1
  Divide1/1 -> Variable Transport Delay1/2
  Divide/1 -> Variable Transport Delay/2
  Sin 2*pi*hr/n./1(sin) -> Product1/2
  Beta/1 -> Variable Transport Delay1/1
  Variable Transport Delay1/1 -> Product1/1
  Variable Transport Delay/1 -> Product/1
  Cos 2*pi*hr/n/1(cos) -> Product/2

== system MDSC_PLL/MDSC_n/MDSC_n/DSC_alpha/Delay 11 ==
  note: Delay Output 11
  Alpha : Inport
  Beta : Inport  Port=2
  1/n : Constant  Value=11/n
  1/n. : Constant  Value=11/n
  Cos 2*pi*hr/n : Subsystem
  Divide : Product  Inputs=*/
  Divide1 : Product  Inputs=*/
  Product : Product
  Product1 : Product
  Sin 2*pi*hr/n. : Subsystem
  Sum : Sum  Inputs=|+-
  Variable Transport Delay : VariableTransportDelay  VariableDelayType=Variable transport delay  MaximumDelay=10
  Variable Transport Delay1 : VariableTransportDelay  VariableDelayType=Variable transport delay  MaximumDelay=10
  DO11 : Outport
  wires:
  Cos 2*pi*hr/n/1(cos) -> Product/2
  Variable Transport Delay/1 -> Product/1
  Variable Transport Delay1/1 -> Product1/1
  Beta/1 -> Variable Transport Delay1/1
  Sin 2*pi*hr/n./1(sin) -> Product1/2
  Divide/1 -> Variable Transport Delay/2
  Divide1/1 -> Variable Transport Delay1/2
  1/n./1 -> Divide1/1
  [f_pll_m3] -> Divide1/2
  [f_pll_m3] -> Divide/2
  1/n/1 -> Divide/1
  Alpha/1 -> Variable Transport Delay/1
  Product/1 -> Sum/1
  Product1/1 -> Sum/2
  Sum/1 -> DO11/1

== system MDSC_PLL/MDSC_n/MDSC_n/DSC_alpha/Delay 12 ==
  note: Delay Output 12
  Alpha : Inport
  Beta : Inport  Port=2
  1/n : Constant  Value=12/n
  1/n. : Constant  Value=12/n
  Cos 2*pi*hr/n : Subsystem
  Divide : Product  Inputs=*/
  Divide1 : Product  Inputs=*/
  Product : Product
  Product1 : Product
  Sin 2*pi*hr/n. : Subsystem
  Sum : Sum  Inputs=|+-
  Variable Transport Delay : VariableTransportDelay  VariableDelayType=Variable transport delay  MaximumDelay=10
  Variable Transport Delay1 : VariableTransportDelay  VariableDelayType=Variable transport delay  MaximumDelay=10
  DO12 : Outport
  wires:
  Sum/1 -> DO12/1
  Product1/1 -> Sum/2
  Product/1 -> Sum/1
  Alpha/1 -> Variable Transport Delay/1
  1/n/1 -> Divide/1
  [f_pll_m3] -> Divide/2
  [f_pll_m3] -> Divide1/2
  1/n./1 -> Divide1/1
  Divide1/1 -> Variable Transport Delay1/2
  Divide/1 -> Variable Transport Delay/2
  Sin 2*pi*hr/n./1(sin) -> Product1/2
  Beta/1 -> Variable Transport Delay1/1
  Variable Transport Delay1/1 -> Product1/1
  Variable Transport Delay/1 -> Product/1
  Cos 2*pi*hr/n/1(cos) -> Product/2

== system MDSC_PLL/MDSC_n/MDSC_n/DSC_alpha/Delay 13 ==
  note: Delay Output 13
  Alpha : Inport
  Beta : Inport  Port=2
  1/n : Constant  Value=13/n
  1/n. : Constant  Value=13/n
  Cos 2*pi*hr/n : Subsystem
  Divide : Product  Inputs=*/
  Divide1 : Product  Inputs=*/
  Product : Product
  Product1 : Product
  Sin 2*pi*hr/n. : Subsystem
  Sum : Sum  Inputs=|+-
  Variable Transport Delay : VariableTransportDelay  VariableDelayType=Variable transport delay  MaximumDelay=10
  Variable Transport Delay1 : VariableTransportDelay  VariableDelayType=Variable transport delay  MaximumDelay=10
  DO13 : Outport
  wires:
  Cos 2*pi*hr/n/1(cos) -> Product/2
  Variable Transport Delay/1 -> Product/1
  Variable Transport Delay1/1 -> Product1/1
  Beta/1 -> Variable Transport Delay1/1
  Sin 2*pi*hr/n./1(sin) -> Product1/2
  Divide/1 -> Variable Transport Delay/2
  Divide1/1 -> Variable Transport Delay1/2
  1/n./1 -> Divide1/1
  [f_pll_m3] -> Divide1/2
  [f_pll_m3] -> Divide/2
  1/n/1 -> Divide/1
  Alpha/1 -> Variable Transport Delay/1
  Product/1 -> Sum/1
  Product1/1 -> Sum/2
  Sum/1 -> DO13/1

== system MDSC_PLL/MDSC_n/MDSC_n/DSC_alpha/Delay 14 ==
  note: Delay Output 14
  Alpha : Inport
  Beta : Inport  Port=2
  1/n : Constant  Value=14/n
  1/n. : Constant  Value=14/n
  Cos 2*pi*hr/n : Subsystem
  Divide : Product  Inputs=*/
  Divide1 : Product  Inputs=*/
  Product : Product
  Product1 : Product
  Sin 2*pi*hr/n. : Subsystem
  Sum : Sum  Inputs=|+-
  Variable Transport Delay : VariableTransportDelay  VariableDelayType=Variable transport delay  MaximumDelay=10
  Variable Transport Delay1 : VariableTransportDelay  VariableDelayType=Variable transport delay  MaximumDelay=10
  DO14 : Outport
  wires:
  Sum/1 -> DO14/1
  Product1/1 -> Sum/2
  Product/1 -> Sum/1
  Alpha/1 -> Variable Transport Delay/1
  1/n/1 -> Divide/1
  [f_pll_m3] -> Divide/2
  [f_pll_m3] -> Divide1/2
  1/n./1 -> Divide1/1
  Divide1/1 -> Variable Transport Delay1/2
  Divide/1 -> Variable Transport Delay/2
  Sin 2*pi*hr/n./1(sin) -> Product1/2
  Beta/1 -> Variable Transport Delay1/1
  Variable Transport Delay1/1 -> Product1/1
  Variable Transport Delay/1 -> Product/1
  Cos 2*pi*hr/n/1(cos) -> Product/2

== system MDSC_PLL/MDSC_n/MDSC_n/DSC_alpha/Delay 2 ==
  note: Delay Output 2
  Alpha : Inport
  Beta : Inport  Port=2
  1/n : Constant  Value=2/n
  1/n. : Constant  Value=2/n
  Cos 2*pi*hr/n : Subsystem
  Divide : Product  Inputs=*/
  Divide1 : Product  Inputs=*/
  Product : Product
  Product1 : Product
  SIn 2*pi*hr/n. : Subsystem
  Sum : Sum  Inputs=|+-
  Variable Transport Delay : VariableTransportDelay  VariableDelayType=Variable transport delay  MaximumDelay=10
  Variable Transport Delay1 : VariableTransportDelay  VariableDelayType=Variable transport delay  MaximumDelay=10
  DO2 : Outport
  wires:
  Sum/1 -> DO2/1
  Product1/1 -> Sum/2
  Product/1 -> Sum/1
  Alpha/1 -> Variable Transport Delay/1
  1/n/1 -> Divide/1
  [f_pll_m3] -> Divide/2
  [f_pll_m3] -> Divide1/2
  1/n./1 -> Divide1/1
  Divide1/1 -> Variable Transport Delay1/2
  Divide/1 -> Variable Transport Delay/2
  SIn 2*pi*hr/n./1(sin) -> Product1/2
  Beta/1 -> Variable Transport Delay1/1
  Variable Transport Delay1/1 -> Product1/1
  Variable Transport Delay/1 -> Product/1
  Cos 2*pi*hr/n/1(cos) -> Product/2

== system MDSC_PLL/MDSC_n/MDSC_n/DSC_alpha/Delay 3 ==
  note: Delay Output 3
  Alpha : Inport
  Beta : Inport  Port=2
  1/n : Constant  Value=3/n
  1/n. : Constant  Value=3/n
  Cos 2*pi*hr/n : Subsystem
  Divide : Product  Inputs=*/
  Divide1 : Product  Inputs=*/
  Product : Product
  Product1 : Product
  Sin 2*pi*hr/n. : Subsystem
  Sum : Sum  Inputs=|+-
  Variable Transport Delay : VariableTransportDelay  VariableDelayType=Variable transport delay  MaximumDelay=10
  Variable Transport Delay1 : VariableTransportDelay  VariableDelayType=Variable transport delay  MaximumDelay=10
  DO3 : Outport
  wires:
  Cos 2*pi*hr/n/1(cos) -> Product/2
  Variable Transport Delay/1 -> Product/1
  Variable Transport Delay1/1 -> Product1/1
  Beta/1 -> Variable Transport Delay1/1
  Sin 2*pi*hr/n./1(sin) -> Product1/2
  Divide/1 -> Variable Transport Delay/2
  Divide1/1 -> Variable Transport Delay1/2
  1/n./1 -> Divide1/1
  [f_pll_m3] -> Divide1/2
  [f_pll_m3] -> Divide/2
  1/n/1 -> Divide/1
  Alpha/1 -> Variable Transport Delay/1
  Product/1 -> Sum/1
  Product1/1 -> Sum/2
  Sum/1 -> DO3/1

== system MDSC_PLL/MDSC_n/MDSC_n/DSC_alpha/Delay 4 ==
  note: Delay Output 4
  Alpha : Inport
  Beta : Inport  Port=2
  1/n : Constant  Value=4/n
  1/n. : Constant  Value=4/n
  Cos 2*pi*hr/n : Subsystem
  Divide : Product  Inputs=*/
  Divide1 : Product  Inputs=*/
  Product : Product
  Product1 : Product
  Sin 2*pi*hr/n. : Subsystem
  Sum : Sum  Inputs=|+-
  Variable Transport Delay : VariableTransportDelay  VariableDelayType=Variable transport delay  MaximumDelay=10
  Variable Transport Delay1 : VariableTransportDelay  VariableDelayType=Variable transport delay  MaximumDelay=10
  DO4 : Outport
  wires:
  Sum/1 -> DO4/1
  Product1/1 -> Sum/2
  Product/1 -> Sum/1
  Alpha/1 -> Variable Transport Delay/1
  1/n/1 -> Divide/1
  [f_pll_m3] -> Divide/2
  [f_pll_m3] -> Divide1/2
  1/n./1 -> Divide1/1
  Divide1/1 -> Variable Transport Delay1/2
  Divide/1 -> Variable Transport Delay/2
  Sin 2*pi*hr/n./1(sin) -> Product1/2
  Beta/1 -> Variable Transport Delay1/1
  Variable Transport Delay1/1 -> Product1/1
  Variable Transport Delay/1 -> Product/1
  Cos 2*pi*hr/n/1(cos) -> Product/2

== system MDSC_PLL/MDSC_n/MDSC_n/DSC_alpha/Delay 5 ==
  note: Delay Output 5
  Alpha : Inport
  Beta : Inport  Port=2
  1/n : Constant  Value=5/n
  1/n. : Constant  Value=5/n
  Cos 2*pi*hr/n : Subsystem
  Divide : Product  Inputs=*/
  Divide1 : Product  Inputs=*/
  Product : Product
  Product1 : Product
  Sin 2*pi*hr/n. : Subsystem
  Sum : Sum  Inputs=|+-
  Variable Transport Delay : VariableTransportDelay  VariableDelayType=Variable transport delay  MaximumDelay=10
  Variable Transport Delay1 : VariableTransportDelay  VariableDelayType=Variable transport delay  MaximumDelay=10
  DO5 : Outport
  wires:
  Cos 2*pi*hr/n/1(cos) -> Product/2
  Variable Transport Delay/1 -> Product/1
  Variable Transport Delay1/1 -> Product1/1
  Beta/1 -> Variable Transport Delay1/1
  Sin 2*pi*hr/n./1(sin) -> Product1/2
  Divide/1 -> Variable Transport Delay/2
  Divide1/1 -> Variable Transport Delay1/2
  1/n./1 -> Divide1/1
  [f_pll_m3] -> Divide1/2
  [f_pll_m3] -> Divide/2
  1/n/1 -> Divide/1
  Alpha/1 -> Variable Transport Delay/1
  Product/1 -> Sum/1
  Product1/1 -> Sum/2
  Sum/1 -> DO5/1

== system MDSC_PLL/MDSC_n/MDSC_n/DSC_alpha/Delay 6 ==
  note: Delay Output 6
  Alpha : Inport
  Beta : Inport  Port=2
  1/n : Constant  Value=6/n
  1/n. : Constant  Value=6/n
  Cos 2*pi*hr/n : Subsystem
  Divide : Product  Inputs=*/
  Divide1 : Product  Inputs=*/
  Product : Product
  Product1 : Product
  Sin 2*pi*hr/n. : Subsystem
  Sum : Sum  Inputs=|+-
  Variable Transport Delay : VariableTransportDelay  VariableDelayType=Variable transport delay  MaximumDelay=10
  Variable Transport Delay1 : VariableTransportDelay  VariableDelayType=Variable transport delay  MaximumDelay=10
  DO6 : Outport
  wires:
  Cos 2*pi*hr/n/1(cos) -> Product/2
  Variable Transport Delay/1 -> Product/1
  Variable Transport Delay1/1 -> Product1/1
  Beta/1 -> Variable Transport Delay1/1
  Sin 2*pi*hr/n./1(sin) -> Product1/2
  Divide/1 -> Variable Transport Delay/2
  Divide1/1 -> Variable Transport Delay1/2
  1/n./1 -> Divide1/1
  [f_pll_m3] -> Divide1/2
  [f_pll_m3] -> Divide/2
  1/n/1 -> Divide/1
  Alpha/1 -> Variable Transport Delay/1
  Product/1 -> Sum/1
  Product1/1 -> Sum/2
  Sum/1 -> DO6/1

== system MDSC_PLL/MDSC_n/MDSC_n/DSC_alpha/Delay 7 ==
  note: Delay Output 7
  Alpha : Inport
  Beta : Inport  Port=2
  1/n : Constant  Value=7/n
  1/n. : Constant  Value=7/n
  Cos 2*pi*hr/n : Subsystem
  Divide : Product  Inputs=*/
  Divide1 : Product  Inputs=*/
  Product : Product
  Product1 : Product
  Sin 2*pi*hr/n. : Subsystem
  Sum : Sum  Inputs=|+-
  Variable Transport Delay : VariableTransportDelay  VariableDelayType=Variable transport delay  MaximumDelay=10
  Variable Transport Delay1 : VariableTransportDelay  VariableDelayType=Variable transport delay  MaximumDelay=10
  DO7 : Outport
  wires:
  Sum/1 -> DO7/1
  Product1/1 -> Sum/2
  Product/1 -> Sum/1
  Alpha/1 -> Variable Transport Delay/1
  1/n/1 -> Divide/1
  [f_pll_m3] -> Divide/2
  [f_pll_m3] -> Divide1/2
  1/n./1 -> Divide1/1
  Divide1/1 -> Variable Transport Delay1/2
  Divide/1 -> Variable Transport Delay/2
  Sin 2*pi*hr/n./1(sin) -> Product1/2
  Beta/1 -> Variable Transport Delay1/1
  Variable Transport Delay1/1 -> Product1/1
  Variable Transport Delay/1 -> Product/1
  Cos 2*pi*hr/n/1(cos) -> Product/2

== system MDSC_PLL/MDSC_n/MDSC_n/DSC_alpha/Delay 8 ==
  note: Delay Output 8
  Alpha : Inport
  Beta : Inport  Port=2
  1/n : Constant  Value=8/n
  1/n. : Constant  Value=8/n
  Cos 2*pi*hr/n : Subsystem
  Divide : Product  Inputs=*/
  Divide1 : Product  Inputs=*/
  Product : Product
  Product1 : Product
  Sin 2*pi*hr/n. : Subsystem
  Sum : Sum  Inputs=|+-
  Variable Transport Delay : VariableTransportDelay  VariableDelayType=Variable transport delay  MaximumDelay=10
  Variable Transport Delay1 : VariableTransportDelay  VariableDelayType=Variable transport delay  MaximumDelay=10
  DO8 : Outport
  wires:
  Cos 2*pi*hr/n/1(cos) -> Product/2
  Variable Transport Delay/1 -> Product/1
  Variable Transport Delay1/1 -> Product1/1
  Beta/1 -> Variable Transport Delay1/1
  Sin 2*pi*hr/n./1(sin) -> Product1/2
  Divide/1 -> Variable Transport Delay/2
  Divide1/1 -> Variable Transport Delay1/2
  1/n./1 -> Divide1/1
  [f_pll_m3] -> Divide1/2
  [f_pll_m3] -> Divide/2
  1/n/1 -> Divide/1
  Alpha/1 -> Variable Transport Delay/1
  Product/1 -> Sum/1
  Product1/1 -> Sum/2
  Sum/1 -> DO8/1

== system MDSC_PLL/MDSC_n/MDSC_n/DSC_alpha/Delay 9 ==
  note: Delay Output 9
  Alpha : Inport
  Beta : Inport  Port=2
  1/n : Constant  Value=9/n
  1/n. : Constant  Value=9/n
  Cos 2*pi*hr/n : Subsystem
  Divide : Product  Inputs=*/
  Divide1 : Product  Inputs=*/
  Product : Product
  Product1 : Product
  Sin 2*pi*hr/n. : Subsystem
  Sum : Sum  Inputs=|+-
  Variable Transport Delay : VariableTransportDelay  VariableDelayType=Variable transport delay  MaximumDelay=10
  Variable Transport Delay1 : VariableTransportDelay  VariableDelayType=Variable transport delay  MaximumDelay=10
  DO9 : Outport
  wires:
  Cos 2*pi*hr/n/1(cos) -> Product/2
  Variable Transport Delay/1 -> Product/1
  Variable Transport Delay1/1 -> Product1/1
  Beta/1 -> Variable Transport Delay1/1
  Sin 2*pi*hr/n./1(sin) -> Product1/2
  Divide/1 -> Variable Transport Delay/2
  Divide1/1 -> Variable Transport Delay1/2
  1/n./1 -> Divide1/1
  [f_pll_m3] -> Divide1/2
  [f_pll_m3] -> Divide/2
  1/n/1 -> Divide/1
  Alpha/1 -> Variable Transport Delay/1
  Product/1 -> Sum/1
  Product1/1 -> Sum/2
  Sum/1 -> DO9/1

== system MDSC_PLL/MDSC_n/MDSC_n/DSC_Beta/Delay 1/Cos 2*pi*hr//n ==
  note: 2*pi*hr/n
  Constant : Constant  Value=2*pi*hr/n
  Trigonometric Function : Trigonometry  Operator=cos
  cos : Outport
  wires:
  Constant/1 -> Trigonometric Function/1
  Trigonometric Function/1 -> cos/1

== system MDSC_PLL/MDSC_n/MDSC_n/DSC_Beta/Delay 1/Sin 2*pi*hr//n. ==
  note: 2*pi*hr/n
  Constant : Constant  Value=2*pi*hr/n
  Trigonometric Function : Trigonometry
  sin : Outport
  wires:
  Constant/1 -> Trigonometric Function/1
  Trigonometric Function/1 -> sin/1

== system MDSC_PLL/MDSC_n/MDSC_n/DSC_Beta/Delay 10/Cos 2*pi*hr//n ==
  note: 2*pi*hr/n
  Constant : Constant  Value=2*pi*hr*10/n
  Trigonometric Function : Trigonometry  Operator=cos
  cos : Outport
  wires:
  Trigonometric Function/1 -> cos/1
  Constant/1 -> Trigonometric Function/1

== system MDSC_PLL/MDSC_n/MDSC_n/DSC_Beta/Delay 10/Sin 2*pi*hr//n. ==
  note: 2*pi*hr/n
  Constant : Constant  Value=2*pi*hr*10/n
  Trigonometric Function : Trigonometry
  sin : Outport
  wires:
  Trigonometric Function/1 -> sin/1
  Constant/1 -> Trigonometric Function/1

== system MDSC_PLL/MDSC_n/MDSC_n/DSC_Beta/Delay 11/Cos 2*pi*hr//n ==
  note: 2*pi*hr/n
  Constant : Constant  Value=2*pi*hr*11/n
  Trigonometric Function : Trigonometry  Operator=cos
  cos : Outport
  wires:
  Constant/1 -> Trigonometric Function/1
  Trigonometric Function/1 -> cos/1

== system MDSC_PLL/MDSC_n/MDSC_n/DSC_Beta/Delay 11/SIn 2*pi*hr//n. ==
  note: 2*pi*hr/n
  Constant : Constant  Value=2*pi*hr*11/n
  Trigonometric Function : Trigonometry
  sin : Outport
  wires:
  Constant/1 -> Trigonometric Function/1
  Trigonometric Function/1 -> sin/1

== system MDSC_PLL/MDSC_n/MDSC_n/DSC_Beta/Delay 12/Cos 2*pi*hr//n ==
  note: 2*pi*hr/n
  Constant : Constant  Value=2*pi*hr*12/n
  Trigonometric Function : Trigonometry  Operator=cos
  cos : Outport
  wires:
  Trigonometric Function/1 -> cos/1
  Constant/1 -> Trigonometric Function/1

== system MDSC_PLL/MDSC_n/MDSC_n/DSC_Beta/Delay 12/Sin 2*pi*hr//n. ==
  note: 2*pi*hr/n
  Constant : Constant  Value=2*pi*hr*12/n
  Trigonometric Function : Trigonometry
  sin : Outport
  wires:
  Trigonometric Function/1 -> sin/1
  Constant/1 -> Trigonometric Function/1

== system MDSC_PLL/MDSC_n/MDSC_n/DSC_Beta/Delay 13/Cos 2*pi*hr//n ==
  note: 2*pi*hr/n
  Constant : Constant  Value=2*pi*hr*13/n
  Trigonometric Function : Trigonometry  Operator=cos
  cos : Outport
  wires:
  Constant/1 -> Trigonometric Function/1
  Trigonometric Function/1 -> cos/1

== system MDSC_PLL/MDSC_n/MDSC_n/DSC_Beta/Delay 13/Sin 2*pi*hr//n. ==
  note: 2*pi*hr/n
  Constant : Constant  Value=2*pi*hr*13/n
  Trigonometric Function : Trigonometry
  sin : Outport
  wires:
  Constant/1 -> Trigonometric Function/1
  Trigonometric Function/1 -> sin/1

== system MDSC_PLL/MDSC_n/MDSC_n/DSC_Beta/Delay 14/Cos 2*pi*hr//n ==
  note: 2*pi*hr/n
  Constant : Constant  Value=2*pi*hr*14/n
  Trigonometric Function : Trigonometry  Operator=cos
  cos : Outport
  wires:
  Trigonometric Function/1 -> cos/1
  Constant/1 -> Trigonometric Function/1

== system MDSC_PLL/MDSC_n/MDSC_n/DSC_Beta/Delay 14/Sin 2*pi*hr//n. ==
  note: 2*pi*hr/n
  Constant : Constant  Value=2*pi*hr*14/n
  Trigonometric Function : Trigonometry
  sin : Outport
  wires:
  Trigonometric Function/1 -> sin/1
  Constant/1 -> Trigonometric Function/1

== system MDSC_PLL/MDSC_n/MDSC_n/DSC_Beta/Delay 2/Cos 2*pi*hr//n ==
  note: 2*pi*hr/n
  Constant : Constant  Value=2*pi*hr*2/n
  Trigonometric Function : Trigonometry  Operator=cos
  cos : Outport
  wires:
  Trigonometric Function/1 -> cos/1
  Constant/1 -> Trigonometric Function/1

== system MDSC_PLL/MDSC_n/MDSC_n/DSC_Beta/Delay 2/Sin 2*pi*hr//n. ==
  note: 2*pi*hr/n
  Constant : Constant  Value=2*pi*hr*2/n
  Trigonometric Function : Trigonometry
  sin : Outport
  wires:
  Trigonometric Function/1 -> sin/1
  Constant/1 -> Trigonometric Function/1

== system MDSC_PLL/MDSC_n/MDSC_n/DSC_Beta/Delay 3/Cos 2*pi*hr//n ==
  note: 2*pi*hr/n
  Constant : Constant  Value=2*pi*hr*3/n
  Trigonometric Function : Trigonometry  Operator=cos
  cos : Outport
  wires:
  Constant/1 -> Trigonometric Function/1
  Trigonometric Function/1 -> cos/1

== system MDSC_PLL/MDSC_n/MDSC_n/DSC_Beta/Delay 3/Sin 2*pi*hr//n. ==
  note: 2*pi*hr/n
  Constant : Constant  Value=2*pi*hr*3/n
  Trigonometric Function : Trigonometry
  sin : Outport
  wires:
  Constant/1 -> Trigonometric Function/1
  Trigonometric Function/1 -> sin/1

== system MDSC_PLL/MDSC_n/MDSC_n/DSC_Beta/Delay 4/Cos 2*pi*hr//n ==
  note: 2*pi*hr/n
  Constant : Constant  Value=2*pi*hr*4/n
  Trigonometric Function : Trigonometry  Operator=cos
  cos : Outport
  wires:
  Trigonometric Function/1 -> cos/1
  Constant/1 -> Trigonometric Function/1

== system MDSC_PLL/MDSC_n/MDSC_n/DSC_Beta/Delay 4/Sin 2*pi*hr//n. ==
  note: 2*pi*hr/n
  Constant : Constant  Value=2*pi*hr*4/n
  Trigonometric Function : Trigonometry
  sin : Outport
  wires:
  Trigonometric Function/1 -> sin/1
  Constant/1 -> Trigonometric Function/1

== system MDSC_PLL/MDSC_n/MDSC_n/DSC_Beta/Delay 5/Cos 2*pi*hr//n ==
  note: 2*pi*hr/n
  Constant : Constant  Value=2*pi*hr*5/n
  Trigonometric Function : Trigonometry  Operator=cos
  cos : Outport
  wires:
  Constant/1 -> Trigonometric Function/1
  Trigonometric Function/1 -> cos/1

== system MDSC_PLL/MDSC_n/MDSC_n/DSC_Beta/Delay 5/Sin 2*pi*hr//n. ==
  note: 2*pi*hr/n
  Constant : Constant  Value=2*pi*hr*5/n
  Trigonometric Function : Trigonometry
  sin : Outport
  wires:
  Constant/1 -> Trigonometric Function/1
  Trigonometric Function/1 -> sin/1

== system MDSC_PLL/MDSC_n/MDSC_n/DSC_Beta/Delay 6/Cos 2*pi*hr//n ==
  note: 2*pi*hr/n
  Constant : Constant  Value=2*pi*hr*6/n
  Trigonometric Function : Trigonometry  Operator=cos
  cos : Outport
  wires:
  Constant/1 -> Trigonometric Function/1
  Trigonometric Function/1 -> cos/1

== system MDSC_PLL/MDSC_n/MDSC_n/DSC_Beta/Delay 6/Sin 2*pi*hr//n. ==
  note: 2*pi*hr/n
  Constant : Constant  Value=2*pi*hr*6/n
  Trigonometric Function : Trigonometry
  sin : Outport
  wires:
  Constant/1 -> Trigonometric Function/1
  Trigonometric Function/1 -> sin/1

== system MDSC_PLL/MDSC_n/MDSC_n/DSC_Beta/Delay 7/Cos 2*pi*hr//n ==
  note: 2*pi*hr/n
  Constant : Constant  Value=2*pi*hr*7/n
  Trigonometric Function : Trigonometry  Operator=cos
  cos : Outport
  wires:
  Trigonometric Function/1 -> cos/1
  Constant/1 -> Trigonometric Function/1
